simulink model "Cook_Tobbe"  (R2018a)
settings: Solver=VariableStepAuto  StartTime=0.0  StopTime=Inf  RelTol=1e-3
libraries: simulink_extras x7
settings Model: Creator=grafton  LastModifiedBy=212454356

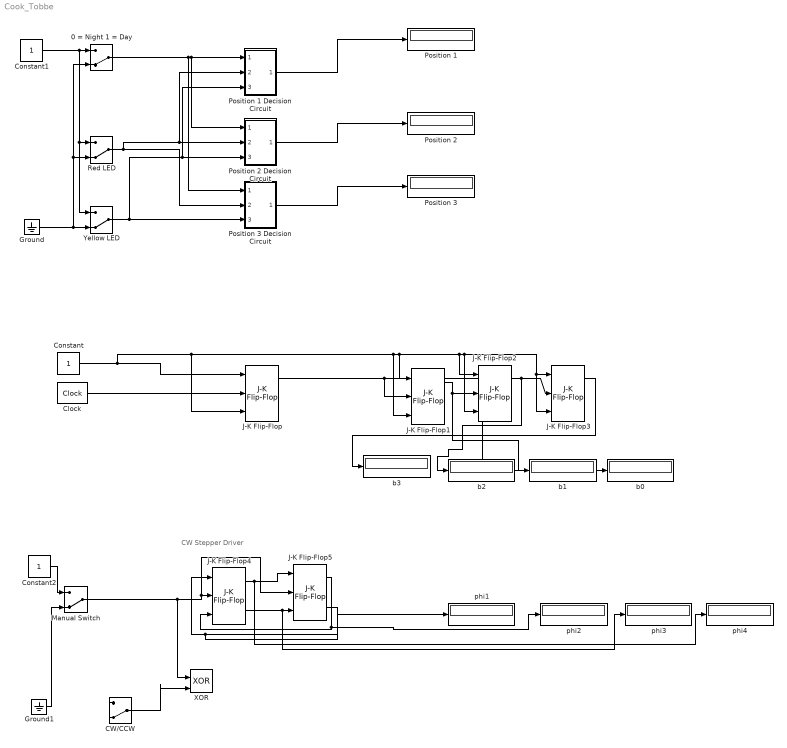
== system Cook_Tobbe ==
  note: CW Stepper Driver
  0 = Night 1 = Day : ManualSwitch  CurrentSetting=0
  CW/CCW : ManualSwitch  CurrentSetting=0
  Clock : simulink_extras/Flip Flops/Clock  period=10
  Constant : Constant  OutDataTypeStr=boolean
  Constant1 : Constant  OutDataTypeStr=boolean
  Constant2 : Constant  OutDataTypeStr=boolean
  Ground : Ground
  Ground1 : Ground
  J-K Flip-Flop{,1..5} (6 alike) : simulink_extras/Flip Flops/J-K Flip-Flop  initial_condition=0
      settings: SourceProductName=Simulink
  Manual Switch : ManualSwitch  CurrentSetting=0
  Position 1 : Display
  Position 1 Decision Circuit : Subsystem
  Position 2 : Display
  Position 2 Decision Circuit : Subsystem
  Position 3 : Display
  Position 3 Decision Circuit : Subsystem
  Red LED : ManualSwitch  CurrentSetting=0
  XOR : Logic  Operator=XOR  IconShape=distinctive  AllPortsSameDT=off  OutDataTypeStr=boolean
  Yellow LED : ManualSwitch  CurrentSetting=0
  b{0..3} (4 alike) : Display
  phi{1..4} (4 alike) : Display
  wires:
  Constant1/1 -> Red LED/1, Yellow LED/1, 0 = Night 1 = Day/1
  Ground/1 -> 0 = Night 1 = Day/2, Red LED/2, Yellow LED/2
  0 = Night 1 = Day/1 -> Position 3 Decision Circuit/1(In1), Position 2 Decision Circuit/1(In1), Position 1 Decision Circuit/1(In1)
  Red LED/1 -> Position 1 Decision Circuit/2(In2), Position 2 Decision Circuit/2(In2), Position 3 Decision Circuit/2(In2)
  Yellow LED/1 -> Position 1 Decision Circuit/3(In3), Position 2 Decision Circuit/3(In3), Position 3 Decision Circuit/3(In3)
  Position 1 Decision Circuit/1(Out1) -> Position 1/1
  Position 2 Decision Circuit/1(Out1) -> Position 2/1
  Position 3 Decision Circuit/1(Out1) -> Position 3/1
  Clock/1 -> J-K Flip-Flop/2
  J-K Flip-Flop/1 -> J-K Flip-Flop1/2, b0/1
  Constant/1 -> J-K Flip-Flop3/3, J-K Flip-Flop3/1, J-K Flip-Flop2/3, J-K Flip-Flop2/1, J-K Flip-Flop1/1, J-K Flip-Flop1/3, J-K Flip-Flop/3, J-K Flip-Flop/1
  J-K Flip-Flop1/1 -> J-K Flip-Flop2/2, b1/1
  J-K Flip-Flop2/1 -> J-K Flip-Flop3/2, b2/1
  J-K Flip-Flop3/1 -> b3/1
  Constant2/1 -> Manual Switch/1
  Ground1/1 -> Manual Switch/2
  J-K Flip-Flop5/1 -> phi2/1, J-K Flip-Flop4/3
  J-K Flip-Flop4/2 -> phi3/1, J-K Flip-Flop5/3
  J-K Flip-Flop4/1 -> phi4/1, J-K Flip-Flop5/1
  J-K Flip-Flop5/2 -> phi1/1, J-K Flip-Flop4/1
  Manual Switch/1 -> XOR/1, J-K Flip-Flop5/2, J-K Flip-Flop4/2
  CW/CCW/1 -> XOR/2

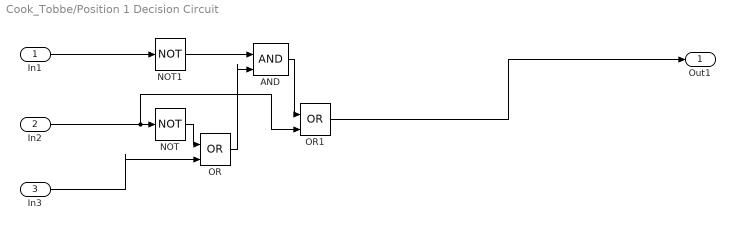
== system Cook_Tobbe/Position 1 Decision Circuit ==
  In1 : Inport
  In2 : Inport  Port=2
  In3 : Inport  Port=3
  AND : Logic  IconShape=distinctive  AllPortsSameDT=off  OutDataTypeStr=boolean
  NOT : Logic  Operator=NOT  IconShape=distinctive  AllPortsSameDT=off  OutDataTypeStr=boolean
  NOT1 : Logic  Operator=NOT  IconShape=distinctive  AllPortsSameDT=off  OutDataTypeStr=boolean
  OR : Logic  Operator=OR  IconShape=distinctive  AllPortsSameDT=off  OutDataTypeStr=boolean
  OR1 : Logic  Operator=OR  IconShape=distinctive  AllPortsSameDT=off  OutDataTypeStr=boolean
  Out1 : Outport
  wires:
  OR/1 -> AND/2
  AND/1 -> OR1/1
  In2/1 -> OR1/2, NOT/1
  NOT/1 -> OR/1
  In1/1 -> NOT1/1
  NOT1/1 -> AND/1
  In3/1 -> OR/2
  OR1/1 -> Out1/1

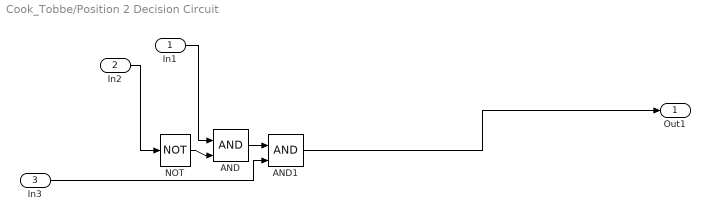
== system Cook_Tobbe/Position 2 Decision Circuit ==
  In1 : Inport
  In2 : Inport  Port=2
  In3 : Inport  Port=3
  AND : Logic  IconShape=distinctive  AllPortsSameDT=off  OutDataTypeStr=boolean
  AND1 : Logic  IconShape=distinctive  AllPortsSameDT=off  OutDataTypeStr=boolean
  NOT : Logic  Operator=NOT  IconShape=distinctive  AllPortsSameDT=off  OutDataTypeStr=boolean
  Out1 : Outport
  wires:
  AND/1 -> AND1/1
  NOT/1 -> AND/2
  In3/1 -> AND1/2
  In2/1 -> NOT/1
  AND1/1 -> Out1/1
  In1/1 -> AND/1

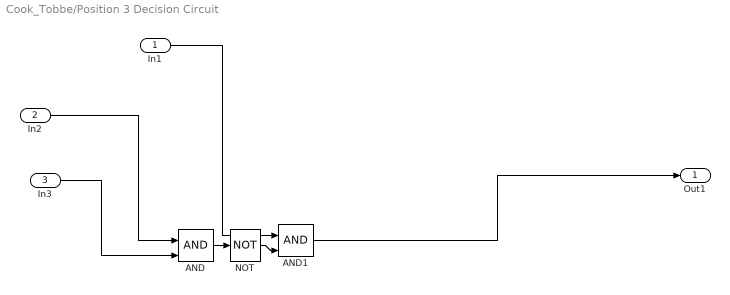
== system Cook_Tobbe/Position 3 Decision Circuit ==
  In1 : Inport
  In2 : Inport  Port=2
  In3 : Inport  Port=3
  AND : Logic  IconShape=distinctive  AllPortsSameDT=off  OutDataTypeStr=boolean
  AND1 : Logic  IconShape=distinctive  AllPortsSameDT=off  OutDataTypeStr=boolean
  NOT : Logic  Operator=NOT  IconShape=distinctive  AllPortsSameDT=off  OutDataTypeStr=boolean
  Out1 : Outport
  wires:
  NOT/1 -> AND1/2
  In3/1 -> AND/2
  In1/1 -> AND1/1
  In2/1 -> AND/1
  AND/1 -> NOT/1
  AND1/1 -> Out1/1
